simulink model "test"  (R2020b)
settings: Solver=VariableStepAuto  StartTime=0.0  StopTime=10.0  RelTol=1e-3
settings Model: Creator=KSL  LastModifiedBy=KSL

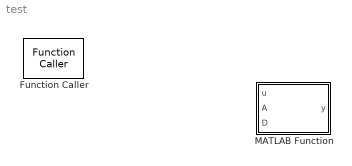
== system test ==
  Function Caller : FunctionCaller  FunctionPrototype=y = f(u)  InputArgumentSpecifications=<Enter example>  OutputArgumentSpecifications=<Enter example>
  MATLAB Function : MATLAB Function  TreatAsAtomicUnit=on

== matlab function test/MATLAB Function ==
  data: u input; y output; A input; D input
function y = fcn(u,A , D)

y = u*A + D;
